simulink model "posture"  (R2022a)
settings: Solver=VariableStepAuto  StartTime=0.0  StopTime=10.0  RelTol=1e-3
settings Model: NumberOfSteps=5  Creator=Lenovo  LastModifiedBy=Lenovo

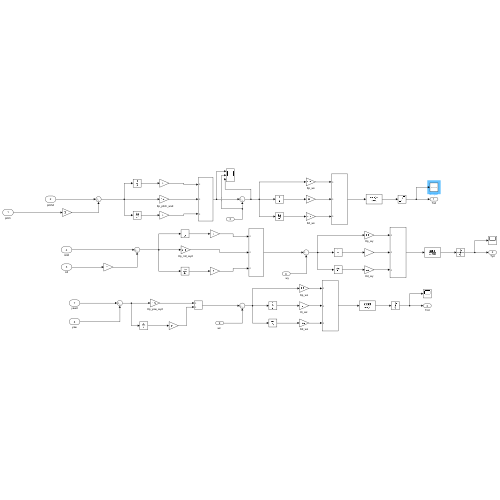
[thumbnail: Simulink's stored preview of the top-level diagram]
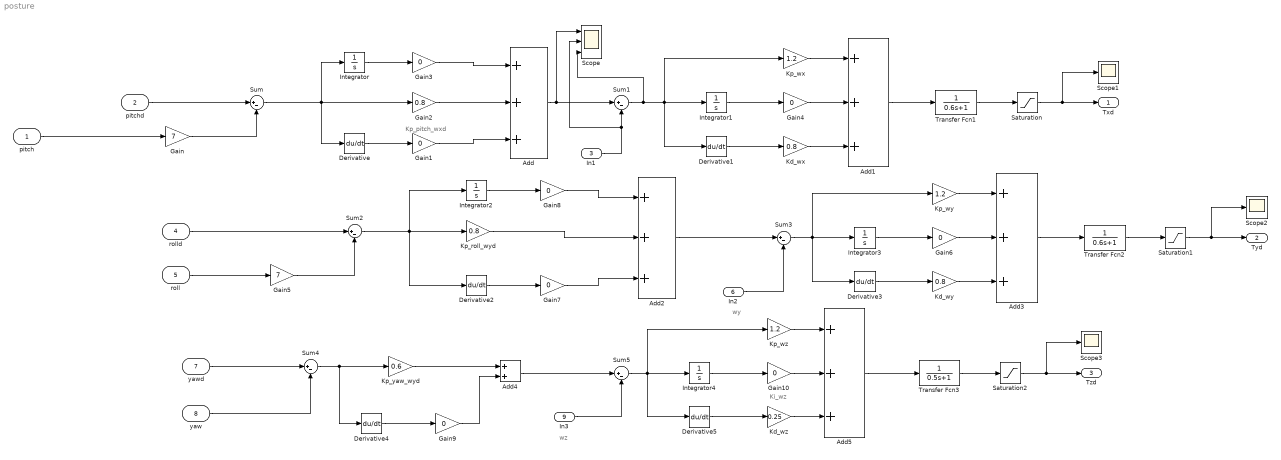
== system posture ==
  note: Ki_wz
  note: wz
  note: wy
  note: Kp_pitch_wxd
  pitch : Inport
  pitchd : Inport  Port=2
  In1 : Inport  Port=3
  rolld : Inport  Port=4
  roll : Inport  Port=5
  In2 : Inport  Port=6
  yawd : Inport  Port=7
  yaw : Inport  Port=8
  In3 : Inport  Port=9
  Add{,1..3,5} (5 alike) : Sum  Inputs=+++
  Add4 : Sum
  Derivative{,1..5} (6 alike) : Derivative
  Gain : Gain  Gain=7
  Gain{1,3..4,6..10} (8 alike) : Gain  Gain=0
  Gain2 : Gain  Gain=0.8
  Gain5 : Gain  Gain=7
  Integrator{,1..4} (5 alike) : Integrator
  Kd_wx : Gain  Gain=0.8
  Kd_wy : Gain  Gain=0.8
  Kd_wz : Gain  Gain=0.25
  Kp_roll_wyd : Gain  Gain=0.8
  Kp_wx : Gain  Gain=1.2
  Kp_wy : Gain  Gain=1.2
  Kp_wz : Gain  Gain=1.2
  Kp_yaw_wyd : Gain  Gain=0.6
  Saturation : Saturate
  Saturation1 : Saturate
  Saturation2 : Saturate
  Scope : Scope  NumInputPorts=3
  Scope1 : Scope
  Scope2 : Scope
  Scope3 : Scope
  Sum{,1..5} (6 alike) : Sum  Inputs=|+-
  Transfer Fcn1 : TransferFcn  Denominator=[0.6 1]
  Transfer Fcn2 : TransferFcn  Denominator=[0.6 1]
  Transfer Fcn3 : TransferFcn  Denominator=[0.5 1]
  Txd : Outport
  Tyd : Outport  Port=2
  Tzd : Outport  Port=3
  wires:
  pitch/1 -> Gain/1
  Gain/1 -> Sum/2
  pitchd/1 -> Sum/1
  Sum/1 -> Gain2/1, Derivative/1, Integrator/1
  Integrator/1 -> Gain3/1
  Derivative/1 -> Gain1/1
  Gain1/1 -> Add/3
  Gain2/1 -> Add/2
  Gain3/1 -> Add/1
  Add/1 -> Scope/1, Sum1/1
  Sum1/1 -> Scope/3, Derivative1/1, Kp_wx/1, Integrator1/1
  Derivative1/1 -> Kd_wx/1
  Integrator1/1 -> Gain4/1
  Gain4/1 -> Add1/2
  Kp_wx/1 -> Add1/1
  Kd_wx/1 -> Add1/3
  Add1/1 -> Transfer Fcn1/1
  Transfer Fcn1/1 -> Saturation/1
  Saturation/1 -> Scope1/1, Txd/1
  In1/1 -> Scope/2, Sum1/2
  Gain5/1 -> Sum2/2
  rolld/1 -> Sum2/1
  Kp_roll_wyd/1 -> Add2/2
  Gain8/1 -> Add2/1
  Gain7/1 -> Add2/3
  Derivative2/1 -> Gain7/1
  Sum2/1 -> Derivative2/1, Integrator2/1, Kp_roll_wyd/1
  Integrator2/1 -> Gain8/1
  Add2/1 -> Sum3/1
  Saturation1/1 -> Tyd/1, Scope2/1
  Transfer Fcn2/1 -> Saturation1/1
  Add3/1 -> Transfer Fcn2/1
  Kd_wy/1 -> Add3/3
  Kp_wy/1 -> Add3/1
  Gain6/1 -> Add3/2
  Integrator3/1 -> Gain6/1
  Derivative3/1 -> Kd_wy/1
  Sum3/1 -> Integrator3/1, Kp_wy/1, Derivative3/1
  In2/1 -> Sum3/2
  roll/1 -> Gain5/1
  yawd/1 -> Sum4/1
  yaw/1 -> Sum4/2
  Sum4/1 -> Derivative4/1, Kp_yaw_wyd/1
  Derivative4/1 -> Gain9/1
  Kp_yaw_wyd/1 -> Add4/1
  Gain9/1 -> Add4/2
  Add4/1 -> Sum5/1
  In3/1 -> Sum5/2
  Sum5/1 -> Derivative5/1, Kp_wz/1, Integrator4/1
  Derivative5/1 -> Kd_wz/1
  Integrator4/1 -> Gain10/1
  Gain10/1 -> Add5/2
  Kp_wz/1 -> Add5/1
  Kd_wz/1 -> Add5/3
  Add5/1 -> Transfer Fcn3/1
  Transfer Fcn3/1 -> Saturation2/1
  Saturation2/1 -> Scope3/1, Tzd/1
